simulink model "exam3_sim"  (R2023a)
settings: Solver=VariableStepAuto  StartTime=0.0  StopTime=5  RelTol=1e-3
values from neighbouring files (symbols this model uses):
  B = 0.0024    [8_21_oct16.mat]    (also in 8_26_oct16.mat; 9_00_oct16_param_wkb.mat; I-PD_pid.mat; exam3.m)
  J_m = 0.005    [8_21_oct16.mat]    (also in 8_26_oct16.mat; 9_00_oct16_param_wkb.mat; I-PD_pid.mat; exam3.m)
  k_i = 1.2879299488    [8_21_oct16.mat]    (also in 8_26_oct16.mat = 1.24340964176; 9_00_oct16_param_wkb.mat = 1.541738552; I-PD_pid.mat = 30; exam3.m = 0.4673766)
  k_p = 4.15772580161    [8_21_oct16.mat]    (also in 8_26_oct16.mat = 9.26358212797; 9_00_oct16_param_wkb.mat = 3.36920723092; I-PD_pid.mat = 3.40616838103; exam3.m = 2.16754540129)
  k_v = omega_0*(2*b_0+k)*J_m-B    (= 0.068418)    [exam3.m]
  M_n = 6.4    [8_21_oct16.mat]    (also in 8_26_oct16.mat; 9_00_oct16_param_wkb.mat; I-PD_pid.mat; exam3.m)
  M_z0 = 0.033    [8_21_oct16.mat]    (also in 8_26_oct16.mat; 9_00_oct16_param_wkb.mat; I-PD_pid.mat; exam3.m)
  Nel = 10000    [8_21_oct16.mat]    (also in 8_26_oct16.mat; 9_00_oct16_param_wkb.mat; I-PD_pid.mat; exam3.m)
  T_n = 0.015    [8_21_oct16.mat]    (also in 8_26_oct16.mat; 9_00_oct16_param_wkb.mat; I-PD_pid.mat; exam3.m)
  Tvz = 0.004    [8_21_oct16.mat]    (also in 8_26_oct16.mat; 9_00_oct16_param_wkb.mat; I-PD_pid.mat; exam3.m)
libraries: SignalEditorBlockLib x1
settings Model: Creator=laptop  LastModifiedBy=laptop

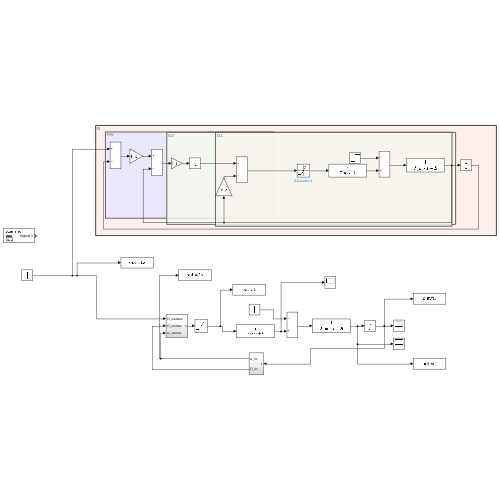
[thumbnail: Simulink's stored preview of the top-level diagram]
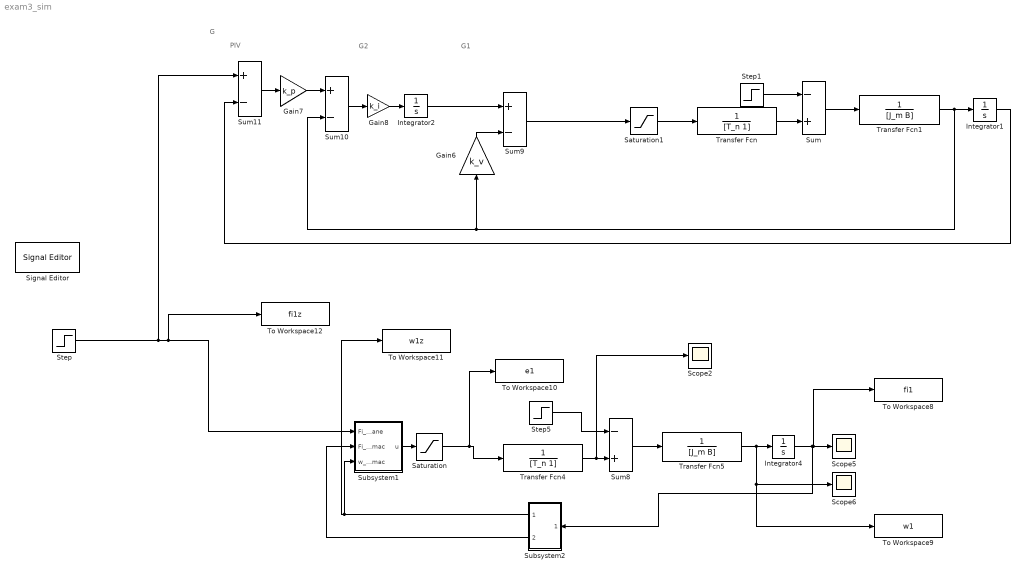
== system exam3_sim ==
  note: G
  note: G2
  note: G1
  note: PIV
  Gain6 : Gain  Gain=k_v
  Gain7 : Gain  Gain=k_p
  Gain8 : Gain  Gain=k_i
  Integrator1 : Integrator
  Integrator2 : Integrator
  Integrator4 : Integrator
  Saturation : Saturate  UpperLimit=M_n*0.75  LowerLimit=-M_n*0.75
  Saturation1 : Saturate  UpperLimit=M_n*0.75  LowerLimit=-M_n*0.75
  Scope2 : Scope
  Scope5 : Scope
  Scope6 : Scope
  Signal Editor : SignalEditorBlockLib/Signal Editor  FileName=signalmat.mat  ActiveScenario=Scenario  ActiveSignal=Signal 1  IsBus=off  OutputBusObjectStr=Bus: BusObject  SampleTime=0  Interpolate=off  ZeroCross=off  OutputAfterFinalValue=Setting to zero  Unit=inherit  PreserveSignalName=on  ApplySigPropsToAllScenarios=on
  Step : Step  Before=pi  After=2*pi  SampleTime=Tvz
  Step1 : Step  Time=3  After=M_z0  SampleTime=0
  Step5 : Step  Time=3  After=M_z0  SampleTime=0
  Subsystem1 : Subsystem
  Subsystem2 : Subsystem
  Sum : Sum  Inputs=-+
  Sum10 : Sum  Inputs=+-
  Sum11 : Sum  Inputs=+-
  Sum8 : Sum  Inputs=-+
  Sum9 : Sum  Inputs=+-
  To Workspace10 : ToWorkspace  VariableName=e1  SaveFormat=Timeseries  SampleTime=-1
  To Workspace11 : ToWorkspace  VariableName=w1z  SaveFormat=Timeseries  SampleTime=-1
  To Workspace12 : ToWorkspace  VariableName=fi1z  SaveFormat=Timeseries  SampleTime=-1
  To Workspace8 : ToWorkspace  VariableName=fi1  SaveFormat=Timeseries  SampleTime=-1
  To Workspace9 : ToWorkspace  VariableName=w1  SaveFormat=Timeseries  SampleTime=-1
  Transfer Fcn : TransferFcn  Denominator=[T_n 1]
  Transfer Fcn1 : TransferFcn  Denominator=[J_m B]
  Transfer Fcn4 : TransferFcn  Denominator=[T_n 1]
  Transfer Fcn5 : TransferFcn  Denominator=[J_m B]
  wires:
  Transfer Fcn/1 -> Sum/2
  Sum/1 -> Transfer Fcn1/1
  Step1/1 -> Sum/1
  Integrator4/1 -> Scope5/1, To Workspace8/1, Subsystem2/1(In1)
  Step5/1 -> Sum8/1
  Transfer Fcn4/1 -> Scope2/1, Sum8/2
  Sum8/1 -> Transfer Fcn5/1
  Transfer Fcn5/1 -> To Workspace9/1, Scope6/1, Integrator4/1
  Subsystem2/2(Fi_irc) -> Subsystem1/2(Fi_snimac)
  Subsystem1/1(u) -> Saturation/1
  Subsystem2/1(w_irc) -> To Workspace11/1, Subsystem1/3(w_snimac)
  Saturation/1 -> Transfer Fcn4/1, To Workspace10/1
  Saturation1/1 -> Transfer Fcn/1
  Sum9/1 -> Saturation1/1
  Transfer Fcn1/1 -> Sum10/2, Gain6/1, Integrator1/1
  Step/1 -> To Workspace12/1, Subsystem1/1(Fi_ziadane), Sum11/1
  Sum11/1 -> Gain7/1
  Integrator2/1 -> Sum9/1
  Gain8/1 -> Integrator2/1
  Integrator1/1 -> Sum11/2
  Gain7/1 -> Sum10/1
  Sum10/1 -> Gain8/1
  Gain6/1 -> Sum9/2

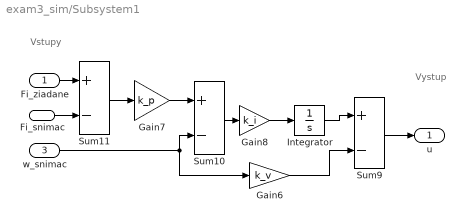
== system exam3_sim/Subsystem1 ==
  note: Vystup
  note: Vstupy
  Fi_ziadane : Inport
  Fi_snimac : Inport  Port=2
  w_snimac : Inport  Port=3
  Gain6 : Gain  Gain=k_v
  Gain7 : Gain  Gain=k_p
  Gain8 : Gain  Gain=k_i
  Integrator : Integrator
  Sum10 : Sum  Inputs=+-
  Sum11 : Sum  Inputs=+-
  Sum9 : Sum  Inputs=+-
  u : Outport
  wires:
  Gain6/1 -> Sum9/2
  Sum10/1 -> Gain8/1
  Gain7/1 -> Sum10/1
  Fi_snimac/1 -> Sum11/2
  Sum9/1 -> u/1
  Sum11/1 -> Gain7/1
  Fi_ziadane/1 -> Sum11/1
  w_snimac/1 -> Gain6/1, Sum10/2
  Gain8/1 -> Integrator/1
  Integrator/1 -> Sum9/1

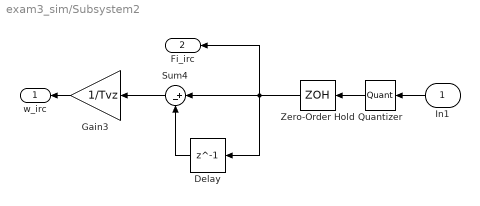
== system exam3_sim/Subsystem2 ==
  In1 : Inport
  Delay : Delay  DelayLength=1
  Gain3 : Gain  Gain=1/Tvz
  Quantizer : Quantizer  QuantizationInterval=2*pi/Nel
  Sum4 : Sum  Inputs=|+-
  Zero-Order Hold : ZeroOrderHold  SampleTime=Tvz
  w_irc : Outport
  Fi_irc : Outport  Port=2
  wires:
  Sum4/1 -> Gain3/1
  Delay/1 -> Sum4/2
  Zero-Order Hold/1 -> Delay/1, Sum4/1, Fi_irc/1
  In1/1 -> Quantizer/1
  Quantizer/1 -> Zero-Order Hold/1
  Gain3/1 -> w_irc/1
